simulink model "beluga1_model_yaw"  (R2016b)
settings: Solver=ode45  StartTime=0.0  StopTime=12  RelTol=1e-8  AbsTol=1e-10
values from neighbouring files (symbols this model uses):
  B = 0.55    [phasePD.m]    (also in run_yaw.m; run_yaw_trials.m; spline_vel.m = [vo; vf; ao; af]; spline_yaw.m = [phi_o; phi_f; ro; rf; ao; af])
  Kd = double(real(Kd.Kd))    [phasePD.m]    (also in run_yaw.m = 3.47)
  Kp = 1.2/A    [calculate_PID.m]    (also in phasePD.m = double(real(Kp)); run_yaw.m = 2.17)
  r_set = pi/2    (= 1.57079632679)    [run_yaw.m]    (also in run_yaw_trials.m)
  tdyaw = 0.11    [run_yaw.m]    (also in run_yaw_trials.m)
settings Model: Creator=bright  LastModifiedBy=omaha
settings DataIOCC: SaveFormat=Array  SignalLoggingSaveFormat=ModelDataLogs  Refine=10
settings OptimizationCC: BlockReduction=off  BooleanDataType=off
settings DebuggingCC: SaveWithParameterizedLinksMsg=none  UnderspecifiedInitializationDetection=Classic  MergeDetectMultiDrivingBlocksExec=none  SignalResolutionControl=TryResolveAllWithWarning  MultiTaskDSMMsg=warning  MultiTaskCondExecSysMsg=none
settings HardwareCC: TargetUnknown=on
settings ModelReferenceCC: PropagateSignalLabelsOutOfModel=off
settings GRTTargetCC: TargetLangStandard=C89/C90 (ANSI)  CombineOutputUpdateFcns=off  GRTInterface=on

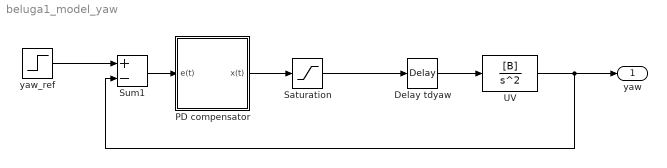
== system beluga1_model_yaw ==
  Delay tdyaw : TransportDelay  DelayTime=tdyaw
  PD compensator : Subsystem
  Saturation : Saturate  UpperLimit=1  LowerLimit=-1  LinearizeAsGain=off  ZeroCross=off
  Sum1 : Sum  Inputs=+-  SaturateOnIntegerOverflow=on  InputSameDT=on  OutDataTypeStr=Inherit: Same as first input
  UV : TransferFcn  Numerator=[B]  Denominator=[1 0 0]
  yaw_ref : Step  Time=0  After=r_set  SampleTime=.001
  yaw : Outport
  wires:
  Delay tdyaw/1 -> UV/1
  yaw_ref/1 -> Sum1/1
  UV/1 -> yaw/1, Sum1/2
  Sum1/1 -> PD compensator/1(e(t))
  PD compensator/1(x(t)) -> Saturation/1
  Saturation/1 -> Delay tdyaw/1

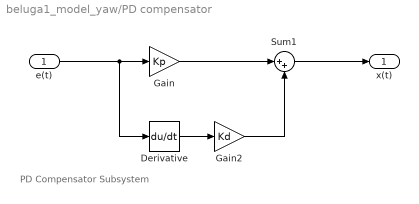
== system beluga1_model_yaw/PD compensator ==
  note: PD Compensator
      | Subsystem
  e(t) : Inport
  Derivative : Derivative
  Gain : Gain  Gain=Kp
  Gain2 : Gain  Gain=Kd
  Sum1 : Sum  Inputs=|++
  x(t) : Outport
  wires:
  Gain2/1 -> Sum1/2
  Gain/1 -> Sum1/1
  Sum1/1 -> x(t)/1
  e(t)/1 -> Gain/1, Derivative/1
  Derivative/1 -> Gain2/1
